simulink model "ship_2d_cartesian"  (R2021b)
settings: Solver=VariableStepAuto  StartTime=0.0  StopTime=10.0  RelTol=1e-3
settings Model: Creator=cirie  LastModifiedBy=cirie

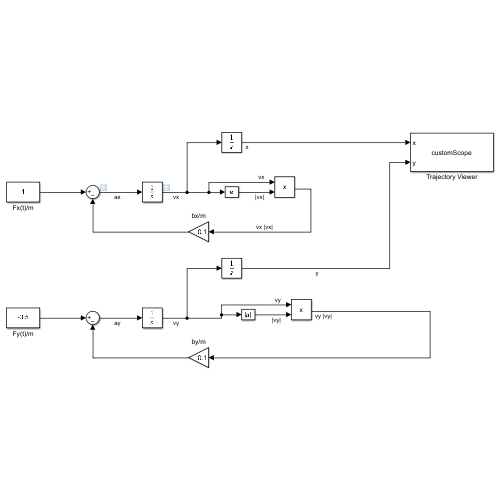
[thumbnail: Simulink's stored preview of the top-level diagram]
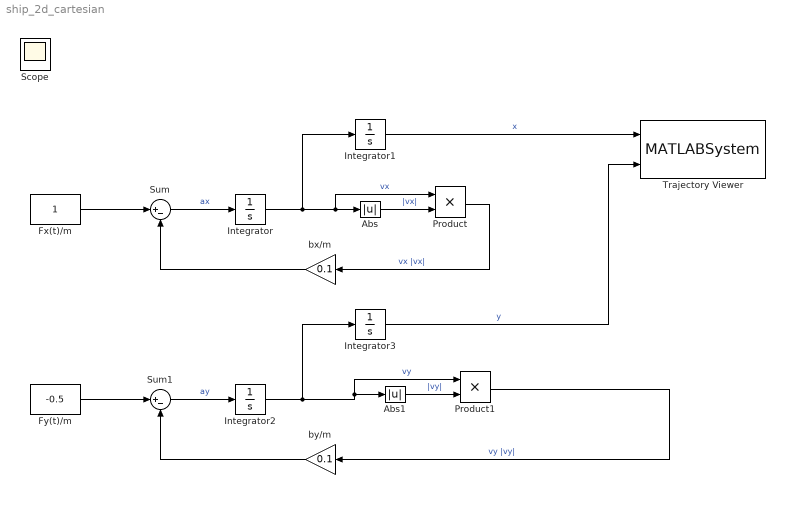
== system ship_2d_cartesian ==
  Abs : Abs
  Abs1 : Abs
  Fx(t)/m : Constant
  Fy(t)/m : Constant  Value=-0.5
  Integrator{,1..3} (4 alike) : Integrator
  Product : Product
  Product1 : Product
  Sum : Sum  Inputs=|+-
  Sum1 : Sum  Inputs=|+-
  Trajectory Viewer : MATLABSystem  System=customScope  fixedAxis=false  xLim=[ -1, 1 ]  yLim=[-1, 1 ]  FigureName=Ship Trajectory  FigureTag=ShipTraj  xLabel=x  yLabel=y  lineColor=[ 0.1843, 0.4941, 0.6980 ]  lineWidth=2
      mask Type: customScope
      mask Display:
      | disp('customScope');
      | port_label('input',1,'x');
      | port_label('input',2,'y');
  bx/m : Gain  Gain=0.1
  by/m : Gain  Gain=0.1
  Scope : Scope
  wires:
  Sum/1 -> Integrator/1  "ax"
  Integrator/1 -> Product/1, Abs/1, Integrator1/1  "vx"
  Product/1 -> bx/m/1  "vx |vx|"
  bx/m/1 -> Sum/2
  Fx(t)/m/1 -> Sum/1
  Fy(t)/m/1 -> Sum1/1
  by/m/1 -> Sum1/2
  Sum1/1 -> Integrator2/1  "ay"
  Integrator1/1 -> Trajectory Viewer/1  "x"
  Integrator3/1 -> Trajectory Viewer/2  "y"
  Abs/1 -> Product/2  "|vx|"
  Integrator2/1 -> Abs1/1, Product1/1, Integrator3/1  "vy"
  Product1/1 -> by/m/1  "vy |vy|"
  Abs1/1 -> Product1/2  "|vy|"
